simulink model "pointing_group24"  (R2023b)
settings: Solver=FixedStepAuto  StartTime=0.0  StopTime=T  RelTol=1e-3
values from neighbouring files (symbols this model uses):
  a = 6939    [Air_Drag_script.m]    (also in main.m = 6939.063; main_group24.m = 6978)
  AccMagn = 0.5    [main_group24.m]
  AccSunSens = 0.125    [main_group24.m]
  ARW = deg2rad(0.10)    [main_group24.m]
  by = 0.1    [main_group24.m]
  bz = 0.1    [main_group24.m]
  c = 2.99792*10^8    (= 299792000)    [main.m]    (also in main_group24.m = 299792458)
  Cd = 2.2    [main_group24.m]
  e = 0    [Air_Drag_script.m]    (also in main.m = 0.001304; main_group24.m)
  G = [gn, gm, gvali, gsvi]    [main.m]    (also in main_group24.m)
  GyroSampleRate = 10    [main_group24.m]
  H = [hn, hm, hvali, hsvi]    [main.m]    (also in main_group24.m)
  H_0 = ((g1_0^2)+(g1_1^2)+(h1_1^2))^0.5    (= 2.98059244128e-05)    [main_group24.m]
  i = deg2rad(97.5307)    [Air_Drag_script.m]    (also in main.m; main_group24.m = deg2rad(98))
  I_tot = [Ix 0 0; 0 Iy 0; 0 0 Iz]    [data_mass.m]    (also in main_group24.m)
  invI_tot = inv(I_tot)    [data_mass.m]    (also in main_group24.m)
  Ix = J(1,1)    [Air_Drag_script.m]    (also in data_mass.m = 0.0755003333333; main.m = 0.057749855; main_group24.m = 0.0755003333333)
  Iy = J(2,2)    [Air_Drag_script.m]    (also in data_mass.m = 0.0755003333333; main.m = 0.04143542; main_group24.m = 0.0755003333333)
  Iz = J(3,3)    [Air_Drag_script.m]    (also in data_mass.m = 0.055; main.m = 0.024624309; main_group24.m = 0.055)
  k1 = 5e-2    (= 0.05)    [main_group24.m]
  k2 = 2.5e-2    (= 0.025)    [main_group24.m]
  m = [0.1; 0.1; 0.1]    [main.m]    (also in main_group24.m)
  MB = [4; 0.1; 0.1; 0.3]    [main.m]    (also in main_group24.m)
  MMnoise = 15e-9*[1; 1; 1]    [main_group24.m]
  MMSampleRate = 1    [main_group24.m]
  mu = 3.98600433e+5    (= 398600.433)    [main.m]    (also in main_group24.m)
  n = 0.0011    [Air_Drag_script.m]    (also in main.m = sqrt(mu/a^3); main_group24.m = sqrt(mu/a^3))
  n_E = 729.2e-07    (= 7.292e-05)    [main_group24.m]
  om_E = 0.000072921    (= 7.2921e-05)    [main_group24.m]
  P = Fe/c    (= 4.52980041279e-06)    [main_group24.m]
  q0 = [ 1 1 1 1 ]'    [Air_Drag_script.m]    (also in main_group24.m = [0 0 0 1]')
  R_e = 6378    [main.m]    (also in main_group24.m)
  rho_air = 1.65e-13    [Air_Drag_script.m]    (also in main_group24.m = 6.967e-13)
  rho_d_body = 0.1*2/3    (= 0.0666666666667)    [main_group24.m]
  rho_d_sp = 0.1*2/3    (= 0.0666666666667)    [main_group24.m]
  rho_s_body = 0.5    [main_group24.m]
  rho_s_sp = 0.1    [main_group24.m]
  RRW = deg2rad(0.3)    [main_group24.m]
  SP = [1; 0.3; 0.1; 0.01]    [main.m]    (also in main_group24.m = [0.25; 0.1; 0.3; 0.01])
undefined symbols (not defined in the file or in its folder): pan, s1, s2, s3, s4, s5, s6, thrust
libraries: vrlib x25, matrix_library x17, simulink_extras x8, sharedutil x3, simulink x1
(part 1 of 5)
settings Model: Creator=hp  LastModifiedBy=adity

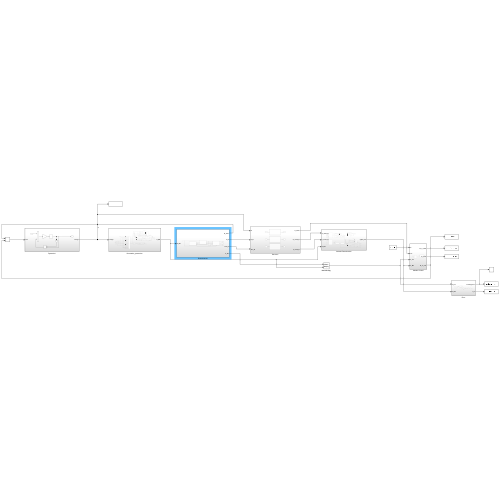
[thumbnail: Simulink's stored preview of the top-level diagram]
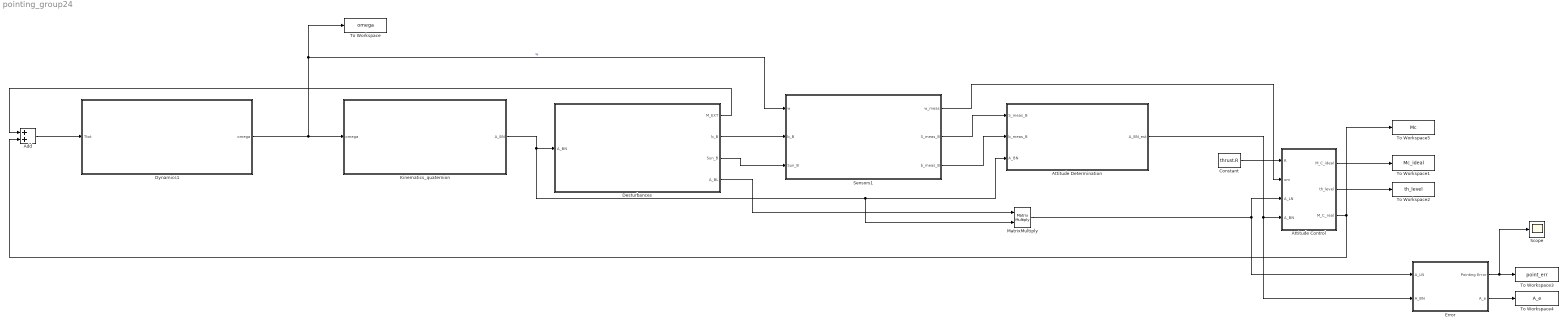
== system pointing_group24 ==
  Add : Sum
  Attitude Control : Subsystem
  Attitude Determination : Subsystem
  Constant : Constant  Value=thrust.R
  Desturbances : Subsystem
  Dynamics1 : Subsystem
  Error : Subsystem
  Kinematics_quaternion : Subsystem
  MatrixMultiply : Product  Multiplication=Matrix(*)
  Scope : Scope
  Sensors1 : Subsystem
  To Workspace : ToWorkspace  VariableName=omega  SaveFormat=Timeseries  SampleTime=-1
  To Workspace1 : ToWorkspace  VariableName=Mc_ideal  SaveFormat=Timeseries  SampleTime=-1
  To Workspace2 : ToWorkspace  VariableName=th_level  SaveFormat=Timeseries  SampleTime=-1
  To Workspace3 : ToWorkspace  VariableName=point_err  SaveFormat=Timeseries  SampleTime=-1
  To Workspace4 : ToWorkspace  VariableName=A_e  SaveFormat=Timeseries  SampleTime=-1
  To Workspace5 : ToWorkspace  VariableName=Mc  SaveFormat=Timeseries  SampleTime=-1
  wires:
  Add/1 -> Dynamics1/1(Ttot)
  Attitude Control/1(M_C_ideal) -> To Workspace1/1
  Attitude Control/2(th_level) -> To Workspace2/1
  Attitude Control/3(M_C_real) -> To Workspace5/1, Add/2
  Desturbances/2(b_B) -> Sensors1/2(b_B)
  Sensors1/2(S_meas_B) -> Attitude Determination/1(S_meas_B)
  Sensors1/1(w_meas) -> Attitude Control/2(om)
  Dynamics1/1(omega) -> Kinematics_quaternion/1(omega), To Workspace/1, Sensors1/1(w)  "w"
  Desturbances/1(M_EXT) -> Add/1
  Sensors1/3(b_meas_B) -> Attitude Determination/2(b_meas_B)
  Desturbances/3(Sun_B) -> Sensors1/3(Sun_B)
  Attitude Determination/1(A_BN_est) -> Error/2(A_BN), Attitude Control/4(A_BN)
  MatrixMultiply/1 -> Attitude Control/3(A_LN), Error/1(A_LN)
  Error/1(Pointing Error) -> Scope/1, To Workspace3/1
  Error/2(A_e) -> To Workspace4/1
  Constant/1 -> Attitude Control/1(R)
  Kinematics_quaternion/1(A_BN) -> MatrixMultiply/2, Attitude Determination/3(A_BN), Desturbances/1(A_BN)
  Desturbances/4(A_BL) -> MatrixMultiply/1

== system pointing_group24/Attitude Control ==
  R : Inport
  om : Inport  Port=2
  A_LN : Inport  Port=3
  A_BN : Inport  Port=4
  Constant : Constant  Value=[0;0;n]
  Ideal controller : Subsystem
  Reshape : Reshape  OutputDimensionality=Column vector (2-D)
  Thrusters : Subsystem
  M_C_ideal : Outport
  th_level : Outport  Port=2
  M_C_real : Outport  Port=3
  wires:
  Constant/1 -> Reshape/1
  Thrusters/3(th_level) -> th_level/1
  om/1 -> Ideal controller/1(om)
  Thrusters/1(M_C_real) -> M_C_real/1
  R/1 -> Thrusters/1(R)
  A_BN/1 -> Ideal controller/3(A_BN)
  Thrusters/2(M_C_ideal) -> M_C_ideal/1
  Ideal controller/1(S) -> Thrusters/2(S)
  Reshape/1 -> Ideal controller/4(om_des)
  A_LN/1 -> Ideal controller/2(A_des)

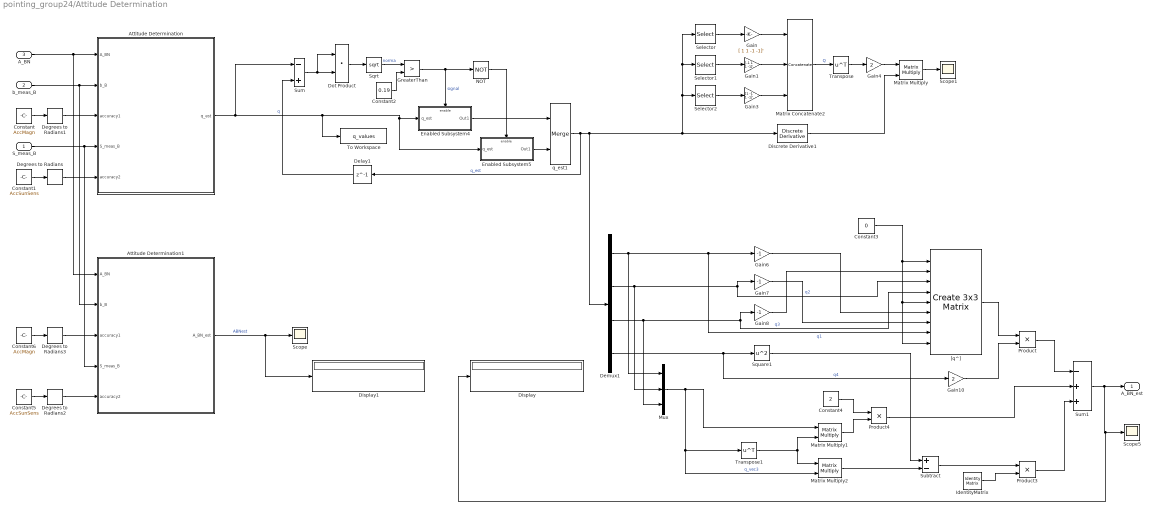
== system pointing_group24/Attitude Determination ==
  S_meas_B : Inport
  b_meas_B : Inport  Port=2
  A_BN : Inport  Port=3
  Attitude Determination : MATLAB Function  TreatAsAtomicUnit=on
  Attitude Determination1 : MATLAB Function  TreatAsAtomicUnit=on
  Constant : Constant  Value=AccMagn
  Constant1 : Constant  Value=AccSunSens
  Constant2 : Constant  Value=0.19
  Constant3 : Constant  Value=0
  Constant4 : Constant  Value=2
  Constant5 : Constant  Value=AccSunSens
  Constant6 : Constant  Value=AccMagn
  Degrees to Radians{,1..3} (4 alike) : simulink_extras/Transformations/Degrees to Radians
  Delay1 : Delay  DelayLength=1  InitialCondition=q0
  Demux1 : Demux
  Discrete Derivative1 : simulink/Discrete/Discrete Derivative  gainval=1.0  ICPrevScaledInput=0  OutMin=[]  OutMax=[]  OutDataType=fixdt(1, 16)  OutScaling=2^-10  DoSatur=off
  Display : Display
  Display1 : Display
  Dot Product : DotProduct  OutDataTypeStr=Inherit: Inherit via internal rule
  Enabled Subsystem4 : Subsystem  TreatAsAtomicUnit=on
  Enabled Subsystem5 : Subsystem  TreatAsAtomicUnit=on
  Gain : Gain  Gain=[ 1 1 -1 -1]'
  Gain1 : Gain  Gain=[-1 1 1 -1]'
  Gain10 : Gain  Gain=2
  Gain3 : Gain  Gain=[1 -1 1 -1]'
  Gain4 : Gain  Gain=2
  Gain6 : Gain  Gain=-1
  Gain7 : Gain  Gain=-1
  Gain8 : Gain  Gain=-1
  GreaterThan : RelationalOperator  Operator=>  OutDataTypeStr=boolean  RndMeth=Simplest  InputSameDT=off
  IdentityMatrix : IdentityMatrix  OutputDimensions=3
  Matrix Concatenate2 : Concatenate  NumInputs=3  Mode=Multidimensional array  ConcatenateDimension=2
  Matrix Multiply : Product  Multiplication=Matrix(*)
  Matrix Multiply1 : Product  Multiplication=Matrix(*)
  Matrix Multiply2 : Product  Multiplication=Matrix(*)
  Mux : Mux  Inputs=3
  NOT : Logic  Operator=NOT  IconShape=distinctive  AllPortsSameDT=off  OutDataTypeStr=boolean
  Product : Product
  Product3 : Product
  Product4 : Product
  Scope : Scope
  Scope1 : Scope
  Scope5 : Scope
  Selector : Selector  InputPortWidth=4  IndexOptions=Index vector (dialog)  Indices=[4 3 2 1]  OutputSizes=1
  Selector1 : Selector  InputPortWidth=4  IndexOptions=Index vector (dialog)  Indices=[3 4 1 2]  OutputSizes=1
  Selector2 : Selector  InputPortWidth=4  IndexOptions=Index vector (dialog)  Indices=[2 1 4 3]  OutputSizes=1
  Sqrt : Sqrt
  Square1 : Math  Operator=square
  Subtract : Sum  Inputs=+-
  Sum : Sum  Inputs=-+
  Sum1 : Sum  Inputs=-++
  To Workspace : ToWorkspace  VariableName=q_values  SaveFormat=Timeseries  SampleTime=-1
  Transpose : Math  Operator=transpose
  Transpose1 : Math  Operator=transpose
  "[q^]" : sharedutil/Create 3x3 Matrix  aMode=aMode
      settings: LibrarySourceBlock=aerolibutil/Create 3x3 Matrix
  q_est1 : Merge
  A_BN_est : Outport
  wires:
  b_meas_B/1 -> Attitude Determination1/2(b_B), Attitude Determination/2(b_B)
  S_meas_B/1 -> Attitude Determination1/4(S_meas_B), Attitude Determination/4(S_meas_B)
  Constant1/1 -> Degrees to Radians/1
  Constant/1 -> Degrees to Radians1/1
  A_BN/1 -> Attitude Determination1/1(A_BN), Attitude Determination/1(A_BN)
  Gain1/1 -> Matrix Concatenate2/2
  Matrix Multiply/1 -> Scope1/1
  Gain4/1 -> Matrix Multiply/1
  Gain/1 -> Matrix Concatenate2/1
  Selector/1 -> Gain/1
  Selector2/1 -> Gain3/1
  Transpose/1 -> Gain4/1
  Discrete Derivative1/1 -> Matrix Multiply/2
  Matrix Concatenate2/1 -> Transpose/1  "Q"
  Selector1/1 -> Gain1/1
  Gain3/1 -> Matrix Concatenate2/3
  Degrees to Radians1/1 -> Attitude Determination/3(accuracy1)
  Degrees to Radians/1 -> Attitude Determination/5(accuracy2)
  q_est1/1 -> Demux1/1, Selector1/1, Selector/1, Selector2/1, Discrete Derivative1/1, Delay1/1  "q_est"
  GreaterThan/1 -> NOT/1, Enabled Subsystem4/Enable  "signal"
  Enabled Subsystem5/1(Out1) -> q_est1/2
  Sum/1 -> Dot Product/1, Dot Product/2
  Delay1/1 -> Sum/2
  NOT/1 -> Enabled Subsystem5/Enable
  Enabled Subsystem4/1(Out1) -> q_est1/1
  Constant2/1 -> GreaterThan/2
  Sqrt/1 -> GreaterThan/1  "norma"
  Dot Product/1 -> Sqrt/1
  Attitude Determination/1(q_est) -> To Workspace/1, Enabled Subsystem4/1(q_est), Enabled Subsystem5/1(q_est), Sum/1  "q"
  "[q^]"/1 -> Product/1
  Square1/1 -> Subtract/1
  Matrix Multiply1/1 -> Product4/2
  Gain10/1 -> Product/2
  Sum1/1 -> Display/1, Scope5/1, A_BN_est/1
  Product/1 -> Sum1/1
  Gain8/1 -> "[q^]"/2
  Constant4/1 -> Product4/1
  Mux/1 -> Matrix Multiply1/1, Transpose1/1, Matrix Multiply2/2  "q_vec3"
  IdentityMatrix/1 -> Product3/2
  Transpose1/1 -> Matrix Multiply1/2, Matrix Multiply2/1
  Matrix Multiply2/1 -> Subtract/2
  Demux1/4 -> Gain10/1, Square1/1  "q4"
  Gain6/1 -> "[q^]"/6
  Demux1/2 -> Mux/2, Gain7/1, "[q^]"/3  "q2"
  Constant3/1 -> "[q^]"/5, "[q^]"/9, "[q^]"/1
  Gain7/1 -> "[q^]"/7
  Demux1/3 -> Mux/3, Gain8/1, "[q^]"/4  "q3"
  Product3/1 -> Sum1/3
  Product4/1 -> Sum1/2
  Demux1/1 -> Mux/1, Gain6/1, "[q^]"/8  "q1"
  Subtract/1 -> Product3/1
  Attitude Determination1/1(A_BN_est) -> Display1/1, Scope/1  "ABNest"
  Degrees to Radians2/1 -> Attitude Determination1/5(accuracy2)
  Constant5/1 -> Degrees to Radians2/1
  Degrees to Radians3/1 -> Attitude Determination1/3(accuracy1)
  Constant6/1 -> Degrees to Radians3/1

== system pointing_group24/Desturbances ==
  A_BN : Inport
  External Torques : Subsystem
      settings: PortSchema="{\"entries\":[{\"content\":{\"sides\":[{\"content\":{\"connectorIds\":[\"In1\",\"In2\",\"In3\",\"In4\",\"In5\"]},\"type\":\"ConnectorPlacement.EquallySpacedRectSide\",\"uuid\":\"8bd06876-b53a-4e9a-80a1-6b2ad32b6751\"},{\"content\":{\"connectorIds\":[\"Out1\",\"Out2\",\"Out3\"],\"side\":\"RIGHT\"},\"type\":\"ConnectorPlacement.EquallySpacedRectSide\",\"uuid\":\"d3d885b4-6948-49f2-a55d-d08402d43087\"},{\"content\":{\"side\":\"TOP\"},\"type\":\"ConnectorPlacement.EquallySpacedRectSide\",\"uuid\":\"3ccb2d92-0b83-4d3b-9d3e-c105f836e6c1\"},{\"content\":{\"connectorIds\":[\"In6\"],\"side\":\"BOTTOM\"},\"type\":\"ConnectorPlacement.EquallySpacedRectSide\",\"uuid\":\"856107a3-6a69-4cc1-b4e3-b2ecd550063c\"}]},\"type\":\"ConnectorPlacement.EquallySpacedConnector\",\"uuid\":\"94a3bf69-72fe-47a3-a305-62b7e77dc891\"}],\"packageUris\":[\"http://schema.mathworks.com/mf0/Connector/R2020b\"],\"version\":\"1.0\"}"
  Orbital Mechanics : Subsystem
  Relative Attitude : Subsystem
  M_EXT : Outport
  b_B : Outport  Port=2
  Sun_B : Outport  Port=3
  A_BL : Outport  Port=4
  wires:
  Relative Attitude/2(r_L) -> External Torques/2(r_L)
  A_BN/1 -> External Torques/5(A_BN), Relative Attitude/1(A_BN_ideal)
  Orbital Mechanics/1(theta) -> Relative Attitude/2(theta)
  Orbital Mechanics/2(r_N) -> Relative Attitude/3(r_N), External Torques/6(r_N)
  Orbital Mechanics/3(r) -> External Torques/3(r)
  External Torques/1(M_EXT) -> M_EXT/1
  External Torques/2(b_B) -> b_B/1
  External Torques/3(Sun_B) -> Sun_B/1
  Orbital Mechanics/4(v_rel_N) -> External Torques/4(v_rel_N)
  Relative Attitude/1(A_BL.) -> A_BL/1, External Torques/1(A_BL)

== system pointing_group24/Dynamics1 ==
  note: omega
  Ttot : Inport
  Add : Sum
  Cross Product : vrlib/Utilities/Cross Product
  Gain : Gain  Gain=invI_tot  Multiplication=Matrix(K*u)
  Gain1 : Gain  Gain=I_tot  Multiplication=Matrix(K*u)
  Integrator3 : Integrator  InitialCondition=[1e-3; 1e-3; 1e-3]  AbsoluteTolerance=10^-7
  omega : Outport
  wires:
  Gain1/1 -> Cross Product/1
  Ttot/1 -> Add/1
  Cross Product/1 -> Add/2
  Integrator3/1 -> omega/1, Cross Product/2, Gain1/1
  Gain/1 -> Integrator3/1
  Add/1 -> Gain/1

== system pointing_group24/Error ==
  A_LN : Inport
  A_BN : Inport  Port=2
  Acos1 : Trigonometry  Operator=acos
  Dot Product : DotProduct  OutDataTypeStr=Inherit: Inherit via internal rule
  Product : Product  Multiplication=Matrix(*)
  Product1 : Product  Multiplication=Matrix(*)
  Radians to Degrees1 : simulink_extras/Transformations/Radians to Degrees
  Transpose : Math  Operator=transpose
  z_B : Constant  Value=[0;0;1]
  z_L : Constant  Value=[0;0;1]
  Pointing Error : Outport
  A_e : Outport  Port=2
  wires:
  A_LN/1 -> Transpose/1
  A_BN/1 -> Product/1
  Transpose/1 -> Product/2
  Product/1 -> Product1/1, A_e/1  "A_BL"
  Radians to Degrees1/1 -> Pointing Error/1
  z_L/1 -> Product1/2
  Dot Product/1 -> Acos1/1
  Acos1/1 -> Radians to Degrees1/1
  Product1/1 -> Dot Product/1  "x_L_B"
  z_B/1 -> Dot Product/2

== system pointing_group24/Kinematics_quaternion ==
  omega : Inport
  Constant : Constant  Value=0
  Constant1 : Constant  Value=0
  Constant2 : Constant  Value=2
  Demux : Demux  Outputs=3
  Demux1 : Demux
  Divide : Product  Inputs=/*
  Dot Product : DotProduct  OutDataTypeStr=Inherit: Inherit via internal rule
  Gain{1..3,6..8} (6 alike) : Gain  Gain=-1
  Gain10 : Gain  Gain=2
  Gain9 : Gain  Gain=1/2
  IdentityMatrix : IdentityMatrix  OutputDimensions=3
  Integrator : Integrator  InitialCondition=q0
  Matrix Multiply : Product  Multiplication=Matrix(*)
  Matrix Multiply1 : Product  Multiplication=Matrix(*)
  Matrix Multiply2 : Product  Multiplication=Matrix(*)
  Mux : Mux  Inputs=3
  OMEGA : Concatenate  NumInputs=16  Mode=Multidimensional array  ConcatenateDimension=2
  Product : Product
  Product3 : Product
  Product4 : Product
  Reshape : Reshape  OutputDimensionality=Customize  OutputDimensions=[4,4]
  Scope : Scope
  Scope5 : Scope
  Square Root2 : Sqrt
  Square1 : Math  Operator=square
  Subtract : Sum  Inputs=+-
  Sum : Sum  Inputs=-++
  Transpose : Math  Operator=transpose
  "[q^]" : sharedutil/Create 3x3 Matrix  aMode=aMode
      settings: LibrarySourceBlock=aerolibutil/Create 3x3 Matrix
  A_BN : Outport
  wires:
  Matrix Multiply/1 -> Gain9/1
  Square Root2/1 -> Divide/1
  Constant/1 -> OMEGA/16, OMEGA/11, OMEGA/6, OMEGA/1
  Integrator/1 -> Dot Product/1, Dot Product/2, Divide/2  "q"
  OMEGA/1 -> Reshape/1
  Constant1/1 -> "[q^]"/5, "[q^]"/9, "[q^]"/1
  Demux1/1 -> Mux/1, Gain6/1, "[q^]"/8  "q1"
  Demux1/2 -> Mux/2, Gain7/1, "[q^]"/3  "q2"
  Demux1/4 -> Gain10/1, Square1/1  "q4"
  Gain8/1 -> "[q^]"/2
  Gain6/1 -> "[q^]"/6
  Gain7/1 -> "[q^]"/7
  Transpose/1 -> Matrix Multiply1/2, Matrix Multiply2/1
  Gain10/1 -> Product/2
  "[q^]"/1 -> Product/1
  Square1/1 -> Subtract/1
  Matrix Multiply2/1 -> Subtract/2
  Divide/1 -> Scope/1, Demux1/1, Matrix Multiply/2  "q"
  Subtract/1 -> Product3/1
  IdentityMatrix/1 -> Product3/2
  Product/1 -> Sum/1
  Product3/1 -> Sum/3
  Constant2/1 -> Product4/1
  Matrix Multiply1/1 -> Product4/2
  Product4/1 -> Sum/2
  Demux1/3 -> Mux/3, Gain8/1, "[q^]"/4  "q3"
  Mux/1 -> Matrix Multiply1/1, Transpose/1, Matrix Multiply2/2  "q_vec3"
  Sum/1 -> Scope5/1, A_BN/1
  Dot Product/1 -> Square Root2/1
  Reshape/1 -> Matrix Multiply/1
  Gain9/1 -> Integrator/1  "q_dot"
  omega/1 -> Demux/1
  Demux/1 -> OMEGA/7, OMEGA/4, Gain2/1  "wx"
  Demux/2 -> OMEGA/8, OMEGA/9, Gain3/1  "wy"
  Demux/3 -> OMEGA/2, OMEGA/12, Gain1/1  "wz"
  Gain3/1 -> OMEGA/3, OMEGA/14
  Gain1/1 -> OMEGA/5, OMEGA/15
  Gain2/1 -> OMEGA/13, OMEGA/10

== system pointing_group24/Sensors1 ==
  w : Inport
  b_B : Inport  Port=2
  Sun_B : Inport  Port=3
  Gyroscope : Subsystem
  Magnetometer : Subsystem
  Sun Sensor : Subsystem
  w_meas : Outport
  S_meas_B : Outport  Port=2
  b_meas_B : Outport  Port=3
  wires:
  w/1 -> Gyroscope/1(w)
  Gyroscope/1(w_meas) -> w_meas/1
  Sun Sensor/1(S_meas_B) -> S_meas_B/1
  Sun_B/1 -> Sun Sensor/1(Sun_B)
  b_B/1 -> Magnetometer/1(b_B)
  Magnetometer/1(b_meas_B) -> b_meas_B/1

== system pointing_group24/Attitude Control/Ideal controller ==
  om : Inport
  A_des : Inport  Port=2
  A_BN : Inport  Port=3
  om_des : Inport  Port=4
  Constant : Constant  Value=[0 0 0]'
  Cross Product : vrlib/Utilities/Cross Product
  Gain : Gain  Gain=I_tot  Multiplication=Matrix(K*u) (u vector)
  Gain1 : Gain  Gain=k1
  Gain2 : Gain  Gain=k2
  Gain4 : Gain  Gain=I_tot  Multiplication=Matrix(K*u) (u vector)
  Gain5 : Gain  Gain=I_tot  Multiplication=Matrix(K*u) (u vector)
  MATLAB Function : MATLAB Function  TreatAsAtomicUnit=on
  Matrix Multiply{1..5} (5 alike) : Product  Multiplication=Matrix(*)
  Subsystem2 : Subsystem
  Sum : Sum
  Sum1 : Sum  Inputs=+-
  Sum2 : Sum  Inputs=-+-
  Sum3 : Sum
  Transpose : Math  Operator=transpose
  S : Outport
  wires:
  Gain1/1 -> Sum/1
  om/1 -> Cross Product/1, Gain/1, Sum1/1
  Matrix Multiply1/1 -> Matrix Multiply2/1, Matrix Multiply5/1, Matrix Multiply3/1, MATLAB Function/1(A)  "A_e"
  Sum1/1 -> Subsystem2/1(om), Gain1/1  "om_e"
  Cross Product/1 -> Sum2/1
  Subsystem2/1(om^) -> Matrix Multiply4/1
  Matrix Multiply2/1 -> Sum1/2
  Matrix Multiply3/1 -> Matrix Multiply4/2
  Gain/1 -> Cross Product/2
  MATLAB Function/1(Av) -> Gain2/1
  Transpose/1 -> Matrix Multiply1/2
  A_BN/1 -> Matrix Multiply1/1
  Sum2/1 -> Sum3/2
  Matrix Multiply4/1 -> Gain4/1
  Matrix Multiply5/1 -> Gain5/1
  A_des/1 -> Transpose/1
  om_des/1 -> Matrix Multiply2/2, Matrix Multiply3/2
  Gain2/1 -> Sum/2
  Sum/1 -> Sum3/1
  Gain4/1 -> Sum2/2
  Gain5/1 -> Sum2/3
  Sum3/1 -> S/1
  Constant/1 -> Matrix Multiply5/2

== system pointing_group24/Attitude Control/Thrusters ==
  R : Inport
  S : Inport  Port=2
  Constant : Constant  Value=thrust.w
  Constant1 : Constant  Value=thrust.T_min
  Constant2 : Constant  Value=thrust.T_max
  Divide : Product  Inputs=*/
  Ideal Control Torque : Subsystem
  MATLAB Function1 : MATLAB Function  TreatAsAtomicUnit=on
  MATLAB Function2 : MATLAB Function  TreatAsAtomicUnit=on
  Matrix Multiply : Product  Multiplication=Matrix(*)
  Matrix Multiply1 : Product  Multiplication=Matrix(*)
  Max of Elements : MinMax  Function=max  ZeroCross=off
  Product : Product
  R1 : InportShadow
  Sum : Sum
  M_C_real : Outport
  M_C_ideal : Outport  Port=2
  th_level : Outport  Port=3
  wires:
  MATLAB Function2/2(th_level) -> th_level/1
  Sum/1 -> MATLAB Function2/1(u_c)  "real"
  Matrix Multiply/1 -> Sum/1, Divide/1
  R1/1 -> Matrix Multiply1/1
  Matrix Multiply1/1 -> M_C_real/1
  MATLAB Function1/1(y) -> Matrix Multiply/1
  R/1 -> MATLAB Function1/1(u)
  Ideal Control Torque/1(M_C_ideal) -> M_C_ideal/1, Matrix Multiply/2
  Max of Elements/1 -> Product/1  "gamma"
  Divide/1 -> Max of Elements/1
  Product/1 -> Sum/2
  Constant/1 -> Product/2, Divide/2  "w"
  MATLAB Function2/1(u_c_real) -> Matrix Multiply1/2  "real"
  S/1 -> Ideal Control Torque/1(S)
  Constant1/1 -> MATLAB Function2/2(T_min)
  Constant2/1 -> MATLAB Function2/3(T_max)

== system pointing_group24/Attitude Determination/Enabled Subsystem4 ==
  q_est : Inport
  Enable : EnablePort
  Gain : Gain  Gain=-1
  Out1 : Outport
  wires:
  q_est/1 -> Gain/1
  Gain/1 -> Out1/1

== system pointing_group24/Attitude Determination/Enabled Subsystem5 ==
  q_est : Inport
  Enable : EnablePort
  Out1 : Outport
  wires:
  q_est/1 -> Out1/1

== system pointing_group24/Desturbances/External Torques ==
  A_BL : Inport
  r_L : Inport  Port=2
  r : Inport  Port=3
  v_rel_N : Inport  Port=4
  A_BN : Inport  Port=5
  r_N : Inport  Port=6
  Air Drag : Subsystem
  Constant : Constant  Value=MB
  Constant1 : Constant  Value=SP
  Constant2 : Constant  Value=MB
  Constant3 : Constant  Value=SP
  M_GG : Subsystem
  Mag field senza fcn : Subsystem
  Magnetic field : Subsystem
  MatrixMultiply : Product  Multiplication=Matrix(*)
  Reflected radiation : Subsystem
  SRP con frecce : Subsystem
  Scope{,1..6} (7 alike) : Scope
  Solar radiation : Subsystem
  Sum of Elements : Sum  Inputs=++++
  Sun position : Subsystem
  To Workspace : ToWorkspace  VariableName=M_GG  SaveFormat=Timeseries  SampleTime=-1
  To Workspace1 : ToWorkspace  VariableName=M_SRP  SaveFormat=Timeseries  SampleTime=-1
  To Workspace2 : ToWorkspace  VariableName=M_MAG  SaveFormat=Timeseries  SampleTime=-1
  M_EXT : Outport
  b_B : Outport  Port=2
  Sun_B : Outport  Port=3
  wires:
  r/1 -> M_GG/2(r)
  Constant/1 -> Solar radiation/2(MB)
  Constant1/1 -> Solar radiation/3(SP)
  A_BN/1 -> Reflected radiation/1(A_BN), Solar radiation/1(A_BN), Magnetic field/2(A_BN), MatrixMultiply/1, Mag field senza fcn/2(A_BN), Sun position/1(A_BN)
  Magnetic field/1(M_MAG) -> Scope2/1, Sum of Elements/3, To Workspace2/1
  Sum of Elements/1 -> M_EXT/1
  A_BL/1 -> M_GG/1(A_BL)
  r_L/1 -> Magnetic field/1(r_L)
  M_GG/1(M_GG1) -> Scope/1, Sum of Elements/1, To Workspace/1
  Solar radiation/1(T_SRP) -> Scope1/1, To Workspace1/1, Sum of Elements/2
  Magnetic field/2(b_B) -> b_B/1
  Solar radiation/2(Sun_B) -> Sun_B/1
  Sun position/1(S_B) -> SRP con frecce/1(S_B)
  Mag field senza fcn/1(T_mag) -> Scope3/1
  MatrixMultiply/1 -> Air Drag/1(v_rel_B)
  Air Drag/1(Tair) -> Scope4/1, Sum of Elements/4
  SRP con frecce/1(Tsrp) -> Scope5/1
  r_N/1 -> Reflected radiation/4(r_N), Mag field senza fcn/1(r_N)
  v_rel_N/1 -> MatrixMultiply/2, Air Drag/2(v_rel_N^2)
  Constant3/1 -> Reflected radiation/3(SP)
  Constant2/1 -> Reflected radiation/2(MB)
  Reflected radiation/1(T_reflect) -> Scope6/1

== system pointing_group24/Desturbances/Orbital Mechanics ==
  Sat Position magnitude : Subsystem
  Sat True Anomaly : Subsystem
  Sat pos & rel vel vectors in inertial frame : Subsystem
  Scope : Scope
  theta : Outport
  r_N : Outport  Port=2
  r : Outport  Port=3
  v_rel_N : Outport  Port=4
  wires:
  Sat True Anomaly/1(theta) -> Sat pos & rel vel vectors in inertial frame/2(theta), theta/1, Sat Position magnitude/1(theta)  "theta"
  Sat Position magnitude/1(r) -> Scope/1, r/1, Sat pos & rel vel vectors in inertial frame/1(r)
  Sat pos & rel vel vectors in inertial frame/1(r_N) -> r_N/1  "r_N"
  Sat pos & rel vel vectors in inertial frame/2(v_rel_N) -> v_rel_N/1

== system pointing_group24/Desturbances/Relative Attitude ==
  A_BN_ideal : Inport
  theta : Inport  Port=2
  r_N : Inport  Port=3
  A_BL : Subsystem
  A_LN : Subsystem
  MatrixMultiply : Product  Multiplication=Matrix(*)
  A_BL. : Outport
  r_L : Outport  Port=2
  wires:
  A_LN/1(A_LN) -> MatrixMultiply/1, A_BL/2(A_LN)
  theta/1 -> A_LN/1(theta)
  A_BN_ideal/1 -> A_BL/1(A_BN)
  A_BL/1(A_BL) -> A_BL./1
  r_N/1 -> MatrixMultiply/2
  MatrixMultiply/1 -> r_L/1

== system pointing_group24/Sensors1/Gyroscope ==
  w : Inport
  ARW : RandomNumber  Variance=(deg2rad(ARW)/sqrt(3600)/sqrt(1/GyroSampleRate))^2*[1;1;1]  SampleTime=1/GyroSampleRate
  Integrator : Integrator
  RRW : RandomNumber  Variance=(deg2rad(RRW)/3600/sqrt(1/GyroSampleRate))^2* [1;1;1]  SampleTime=1/GyroSampleRate
  Sum : Sum  Inputs=+++
  w_meas : Outport
  wires:
  RRW/1 -> Integrator/1  "b_dot"
  ARW/1 -> Sum/2  "n"
  Integrator/1 -> Sum/3  "b"
  Sum/1 -> w_meas/1
  w/1 -> Sum/1

== system pointing_group24/Sensors1/Magnetometer ==
  b_B : Inport
  Constant : Constant  Value=MMnoise
  MatrixMultiply : Product  Multiplication=Matrix(*)
  Subsystem : Subsystem
  Sum : Sum
  b_meas_B : Outport
  wires:
  Constant/1 -> Sum/2
  b_B/1 -> Sum/1  "b_B"
  Subsystem/1(A_epsMM) -> MatrixMultiply/1
  Sum/1 -> MatrixMultiply/2
  MatrixMultiply/1 -> b_meas_B/1

== system pointing_group24/Sensors1/Sun Sensor ==
  Sun_B : Inport
  Matrix Multiply1 : Product  Multiplication=Matrix(*)
  Subsystem : Subsystem
  S_meas_B : Outport
  wires:
  Sun_B/1 -> Matrix Multiply1/2
  Subsystem/1(A_eps) -> Matrix Multiply1/1  "A_eps"
  Matrix Multiply1/1 -> S_meas_B/1

== system pointing_group24/Attitude Control/Ideal controller/Subsystem2 ==
  om : Inport
  Constant : Constant  Value=0
  Demux : Demux  Outputs=3
  Gain : Gain  Gain=-1
  Gain1 : Gain  Gain=-1
  Gain2 : Gain  Gain=-1
  Subsystem : Subsystem
  om^ : Outport
  wires:
  Demux/2 -> Subsystem/3(A13), Gain2/1
  Demux/3 -> Subsystem/4(A21), Gain/1
  Gain2/1 -> Subsystem/7(A31)
  Gain/1 -> Subsystem/2(A12)
  Subsystem/1(A_BN_312) -> om^/1
  Constant/1 -> Subsystem/1(A11), Subsystem/5(A22), Subsystem/9(A33)
  Demux/1 -> Subsystem/8(A32), Gain1/1
  Gain1/1 -> Subsystem/6(A23)
  om/1 -> Demux/1

== system pointing_group24/Attitude Control/Thrusters/Ideal Control Torque ==
  S : Inport
  Constant : Constant  Value=thrust.T_min
  Constant1 : Constant  Value=thrust.T_max
  Constant4 : Constant  Value=[bz;bz;by]
  Gain3 : Gain  Gain=-1
  MATLAB Function2 : MATLAB Function  TreatAsAtomicUnit=on
  Matrix Multiply : Product
  Product2 : Product
  Sign : Signum
  M_C_ideal : Outport
  wires:
  S/1 -> Sign/1, MATLAB Function2/1(S)
  Product2/1 -> Gain3/1
  Gain3/1 -> M_C_ideal/1
  Matrix Multiply/1 -> Product2/1
  MATLAB Function2/1(T) -> Matrix Multiply/2
  Sign/1 -> Product2/2
  Constant4/1 -> Matrix Multiply/1
  Constant/1 -> MATLAB Function2/2(T_min)
  Constant1/1 -> MATLAB Function2/3(T_max)

== system pointing_group24/Desturbances/External Torques/Air Drag ==
  v_rel_B : Inport
  v_rel_N^2 : Inport  Port=2
  Dot Product : DotProduct  OutDataTypeStr=Inherit: Inherit via internal rule
  Gain : Gain  Gain=4
  Gain1 : Gain  Gain=4
  Normalize Vector1 : vrlib/Utilities/Normalize Vector  maxzero=0
  Subsystem : Subsystem
  Subsystem1 : Subsystem
  Subsystem2 : Subsystem
  Subsystem3 : Subsystem
  Subsystem4 : Subsystem
  Subsystem5 : Subsystem
  Subsystem6 : Subsystem
  Subsystem7 : Subsystem
  Sum : Sum  Inputs=++++++++
  Tair : Outport
  wires:
  v_rel_B/1 -> Normalize Vector1/1
  Sum/1 -> Tair/1
  Subsystem/1(Pan1) -> Sum/1
  Subsystem1/1(Pan2) -> Sum/2
  Subsystem2/1(Pan3) -> Sum/3
  Subsystem3/1(Pan4) -> Sum/4
  Subsystem4/1(Pan5) -> Sum/5
  Subsystem5/1(Pan6) -> Sum/6
  Subsystem6/1(Ps1) -> Gain1/1
  Subsystem7/1(Ps2) -> Gain/1
  Gain/1 -> Sum/8
  Gain1/1 -> Sum/7
  Normalize Vector1/1 -> Subsystem1/2(v_rel_B), Subsystem2/2(v_rel_B), Subsystem3/2(v_rel_B), Subsystem4/2(v_rel_B), Subsystem5/2(v_rel_B), Subsystem6/2(v_rel_B), Subsystem7/2(v_rel_B), Subsystem/2(v_rel_B)
  v_rel_N^2/1 -> Dot Product/2, Dot Product/1
  Dot Product/1 -> Subsystem/1(v_rel_N^2), Subsystem1/1(v_rel_N^2), Subsystem2/1(v_rel_N^2), Subsystem3/1(v_rel_N^2), Subsystem4/1(v_rel_N^2), Subsystem5/1(v_rel_N^2), Subsystem6/1(v_rel_N^2), Subsystem7/1(v_rel_N^2)

== system pointing_group24/Desturbances/External Torques/M_GG ==
  A_BL : Inport
  r : Inport  Port=2
  GG Torque1 : Subsystem
  "c1, c2, c3" : Subsystem
  M_GG1 : Outport
  wires:
  A_BL/1 -> "c1, c2, c3"/1(A_BL)
  "c1, c2, c3"/1(c1) -> GG Torque1/1(c1)
  "c1, c2, c3"/2(c2) -> GG Torque1/2(c2)
  "c1, c2, c3"/3(c3) -> GG Torque1/3(c3)
  r/1 -> GG Torque1/4(r)
  GG Torque1/1(M_GG) -> M_GG1/1

== system pointing_group24/Desturbances/External Torques/Mag field senza fcn ==
  r_N : Inport
  A_BN : Inport  Port=2
  Add : Sum  Inputs=-+
  Clock : Clock
  Constant : Constant  Value=11.5
  Constant1 : Constant  Value=n_E
  Constant2 : Constant  Value=H_0
  Constant3 : Constant  Value=R_e
  Constant4 : Constant  Value=3
  Constant5 : Constant  Value=3
  Constant6 : Constant  Value=3
  Constant7 : Constant  Value=m
  Cos : Trigonometry  Operator=cos
  Cos1 : Trigonometry  Operator=cos
  Cross Product : vrlib/Utilities/Cross Product
  Degrees to Radians : simulink_extras/Transformations/Degrees to Radians
  Divide : Product  Inputs=/*
  Dot Product : DotProduct  OutDataTypeStr=Inherit: Inherit via internal rule
  Dot Product1 : DotProduct  OutDataTypeStr=Inherit: Inherit via internal rule
  Gain : Gain  Gain=-1
  MatrixMultiply : Product  Multiplication=Matrix(*)
  Mux : Mux  Inputs=3
  Normalize Vector : vrlib/Utilities/Normalize Vector  maxzero=0
  Power : Math  Operator=pow
  Power1 : Math  Operator=pow
  Product{,1..6} (7 alike) : Product
  Scope : Scope
  Sin : Trigonometry
  Sin1 : Trigonometry
  Sqrt : Sqrt
  T_mag : Outport
  wires:
  Constant/1 -> Degrees to Radians/1
  Constant1/1 -> Product/1
  Clock/1 -> Product/2
  Product/1 -> Sin1/1, Cos/1
  Sin/1 -> Product2/1, Product1/1
  Cos/1 -> Product1/2
  Sin1/1 -> Product2/2
  Product1/1 -> Mux/1
  Cos1/1 -> Mux/3
  Product2/1 -> Mux/2
  Constant4/1 -> Power/2
  Constant3/1 -> Power/1
  Constant5/1 -> Power1/2
  Constant2/1 -> Product3/1
  Power/1 -> Product3/2
  r_N/1 -> Dot Product/2, Dot Product/1, Normalize Vector/1
  Dot Product/1 -> Sqrt/1
  Sqrt/1 -> Power1/1
  Mux/1 -> Gain/1
  Normalize Vector/1 -> Product4/2, Dot Product1/2
  Dot Product1/1 -> Product4/1
  Constant6/1 -> Product5/1
  Product4/1 -> Product5/2
  Product6/1 -> MatrixMultiply/2
  A_BN/1 -> MatrixMultiply/1
  MatrixMultiply/1 -> Cross Product/2
  Constant7/1 -> Cross Product/1
  Cross Product/1 -> Scope/1, T_mag/1
  Product5/1 -> Add/2
  Power1/1 -> Divide/1
  Product3/1 -> Divide/2
  Add/1 -> Product6/1
  Divide/1 -> Product6/2
  Degrees to Radians/1 -> Cos1/1, Sin/1
  Gain/1 -> Dot Product1/1, Add/1

== system pointing_group24/Desturbances/External Torques/Magnetic field ==
  r_L : Inport
  A_BN : Inport  Port=2
  Clock : Clock
  Constant : Constant  Value=m
  Constant1 : Constant  Value=R_e*1000
  Constant3 : Constant  Value=G
  Constant4 : Constant  Value=H
  Cross Product1 : matrix_library/Cross Product
  MATLAB Function : MATLAB Function  TreatAsAtomicUnit=on
  MatrixMultiply : Product  Multiplication=Matrix(*)
  Normalize Vector : vrlib/Utilities/Normalize Vector  maxzero=0
  Reshape1 : Reshape  OutputDimensionality=Column vector (2-D)
  M_MAG : Outport
  b_B : Outport  Port=2
  wires:
  Constant1/1 -> MATLAB Function/2(r)
  Clock/1 -> MATLAB Function/3(t)
  Constant3/1 -> MATLAB Function/4(G)
  MATLAB Function/1(b_N) -> Reshape1/1
  r_L/1 -> MATLAB Function/1(r_LVLH)
  Reshape1/1 -> MatrixMultiply/2
  Constant4/1 -> MATLAB Function/5(H)
  A_BN/1 -> MatrixMultiply/1
  Constant/1 -> Cross Product1/1
  MatrixMultiply/1 -> Normalize Vector/1, Cross Product1/2
  Cross Product1/1 -> M_MAG/1
  Normalize Vector/1 -> b_B/1

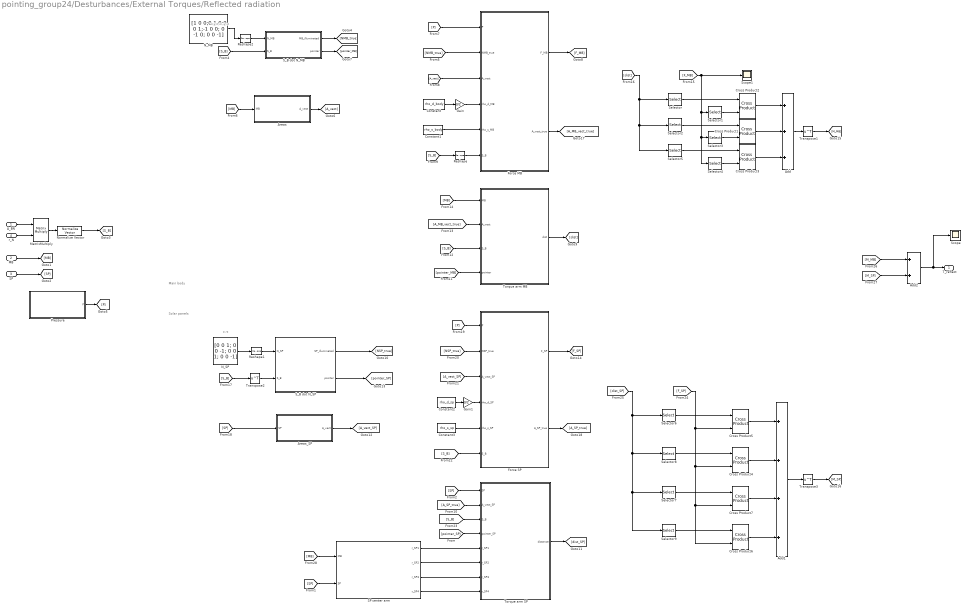
== system pointing_group24/Desturbances/External Torques/Reflected radiation ==
  note: Solar panels
  note: z,-z
  note: x,y,z,-x,-y,-z
  note: Main body
  A_BN : Inport
  MB : Inport  Port=2
  SP : Inport  Port=3
  r_N : Inport  Port=4
  Add : Sum  Inputs=3
  Add1 : Sum  Inputs=++++
  Add2 : Sum
  Areas : Subsystem
  Areas_SP : Subsystem
  Constant : Constant  Value=rho_d_body
  Constant1 : Constant  Value=rho_s_body
  Constant2 : Constant  Value=rho_d_sp
  Constant3 : Constant  Value=rho_s_sp
  Cross Product{1..7} (7 alike) : matrix_library/Cross Product
  Force MB : Subsystem
  Force SP : Subsystem
  Gain : Gain  Gain=3/2
  Gain1 : Gain  Gain=3/2
  MatrixMultiply : Product  Multiplication=Matrix(*)
  N_MB : Constant  Value=[1 0 0;0 1 0;0 0 1;-1 0 0; 0 -1 0; 0 0 -1]  VectorParams1D=off
  N_SP : Constant  Value=[0 0 1; 0 0 -1; 0 0 1; 0 0 -1]  VectorParams1D=off
  Normalize Vector : vrlib/Utilities/Normalize Vector  maxzero=0
  Pressure : Subsystem
  Reshape : Reshape  OutputDimensionality=Column vector (2-D)
  Reshape1 : Reshape  OutputDimensionality=Customize  OutputDimensions=[4,3]
  Reshape2 : Reshape  OutputDimensionality=Customize  OutputDimensions=[6,3]
  SP center arm : Subsystem
  S_B dot N_MB : Subsystem
  S_B dot N_SP : Subsystem
  Scope : Scope
  Scope1 : Scope
  Selector : Selector  NumberOfDimensions=2  InputPortWidth=3  IndexOptions=Index vector (dialog),Index vector (dialog)  Indices=1,[1 2 3]  OutputSizes=1,1
  Selector1 : Selector  NumberOfDimensions=2  InputPortWidth=3  IndexOptions=Index vector (dialog),Index vector (dialog)  Indices=1,[1 2 3]  OutputSizes=1,1
  Selector2 : Selector  NumberOfDimensions=2  InputPortWidth=3  IndexOptions=Index vector (dialog),Index vector (dialog)  Indices=2,[1 2 3]  OutputSizes=1,1
  Selector3 : Selector  NumberOfDimensions=2  InputPortWidth=3  IndexOptions=Index vector (dialog),Index vector (dialog)  Indices=2,[1 2 3]  OutputSizes=1,1
  Selector4 : Selector  NumberOfDimensions=2  InputPortWidth=3  IndexOptions=Index vector (dialog),Index vector (dialog)  Indices=3,[1 2 3]  OutputSizes=1,1
  Selector5 : Selector  NumberOfDimensions=2  InputPortWidth=3  IndexOptions=Index vector (dialog),Index vector (dialog)  Indices=3,[1 2 3]  OutputSizes=1,1
  Selector6 : Selector  NumberOfDimensions=2  InputPortWidth=3  IndexOptions=Index vector (dialog),Index vector (dialog)  Indices=1,[1 2 3]  OutputSizes=1,1
  Selector7 : Selector  NumberOfDimensions=2  InputPortWidth=3  IndexOptions=Index vector (dialog),Index vector (dialog)  Indices=3,[1 2 3]  OutputSizes=1,1
  Selector8 : Selector  NumberOfDimensions=2  InputPortWidth=3  IndexOptions=Index vector (dialog),Index vector (dialog)  Indices=2,[1 2 3]  OutputSizes=1,1
  Selector9 : Selector  NumberOfDimensions=2  InputPortWidth=3  IndexOptions=Index vector (dialog),Index vector (dialog)  Indices=4,[1 2 3]  OutputSizes=1,1
  Torque arm MB : Subsystem
  Torque arm SP : Subsystem
  Transpose1 : Math  Operator=transpose
  Transpose2 : Math  Operator=transpose
  Transpose3 : Math  Operator=transpose
  T_reflect : Outport
  wires:
  Cross Product7/1 -> Add1/3
  Cross Product6/1 -> Add1/4
  [F_SP] -> Cross Product4/2, Cross Product7/2, Cross Product6/2, Cross Product5/2
  [dist_SP] -> Selector8/1, Selector7/1, Selector9/1, Selector6/1
  Selector9/1 -> Cross Product6/1
  Selector7/1 -> Cross Product7/1
  SP center arm/4(r_SP4) -> Torque arm SP/8(r_SP4)
  SP center arm/3(r_SP3) -> Torque arm SP/7(r_SP3)
  Gain1/1 -> Force SP/4(rho_d_SP)
  Gain/1 -> Force MB/4(rho_d_MB)
  SP center arm/2(r_SP2) -> Torque arm SP/6(r_SP2)
  SP center arm/1(r_SP1) -> Torque arm SP/5(r_SP1)
  [MB] -> SP center arm/1(MB)
  [SP] -> SP center arm/2(SP)
  Cross Product3/1 -> Add/3
  [SP] -> Torque arm SP/1(SP)
  [M_SP] -> Add2/2
  Cross Product1/1 -> Add/2
  Selector5/1 -> Cross Product3/1
  Selector6/1 -> Cross Product5/1
  S_B dot N_SP/1(SP_illuminated) -> [NSP_true]
  Force SP/1(F_SP) -> [F_SP]
  Cross Product2/1 -> Add/1
  Reshape/1 -> Force MB/6(S_B)
  [A_vect_SP] -> Force SP/3(A_vect_SP)
  Cross Product5/1 -> Add1/1
  [S_B] -> Transpose2/1
  [S_B] -> Force SP/6(S_B)
  Selector3/1 -> Cross Product1/2
  Add2/1 -> T_reflect/1, Scope/1
  [pointer_MB] -> Torque arm MB/4(pointer)
  Force MB/2(A_vect_true) -> [A_MB_vect_true]
  S_B dot N_MB/2(pointer) -> [pointer_MB]
  Selector4/1 -> Cross Product3/2
  SP/1 -> [SP]
  [S_B] -> Torque arm SP/3(S_B)
  Force SP/2(A_SP_true) -> [A_SP_true]
  [S_B] -> Torque arm MB/3(S_B)
  N_SP/1 -> Reshape1/1
  [NSP_true] -> Force SP/2(NSP_true)
  [dist] -> Selector/1, Selector5/1, Selector2/1
  Selector8/1 -> Cross Product4/1
  Constant/1 -> Gain/1
  Constant2/1 -> Gain1/1
  Normalize Vector/1 -> [S_B]
  Pressure/1(P) -> [P]
  [A_MB_vect_true] -> Torque arm MB/2(A_vect)
  Constant1/1 -> Force MB/5(rho_s_MB)
  Selector1/1 -> Cross Product2/2
  [A_vect] -> Force MB/3(A_vect)
  [P] -> Force SP/1(P)
  [S_B] -> Reshape/1
  Selector/1 -> Cross Product2/1
  Force MB/1(F_MB) -> [F_MB]
  S_B dot N_SP/2(pointer) -> [pointer_SP]
  Torque arm MB/1(dist) -> [dist]
  Reshape2/1 -> S_B dot N_MB/1(N_MB)
  Torque arm SP/1(distance) -> [dist_SP]
  Add/1 -> Transpose1/1
  [A_SP_true] -> Torque arm SP/2(A_vect_SP)
  [SP] -> Areas_SP/1(SP)
  Transpose2/1 -> S_B dot N_SP/2(S_B)
  Add1/1 -> Transpose3/1
  A_BN/1 -> MatrixMultiply/1
  [F_MB] -> Selector1/1, Selector3/1, Selector4/1, Scope1/1
  Cross Product4/1 -> Add1/2
  [pointer_SP] -> Torque arm SP/4(pointer_SP)
  [M_MB] -> Add2/1
  Constant3/1 -> Force SP/5(rho_s_SP)
  [MB] -> Torque arm MB/1(MB)
  Selector2/1 -> Cross Product1/1
  Transpose3/1 -> [M_SP]
  Reshape1/1 -> S_B dot N_SP/1(N_SP)
  Areas_SP/1(A_vect) -> [A_vect_SP]
  Transpose1/1 -> [M_MB]
  Areas/1(A_vect) -> [A_vect]
  [P] -> Force MB/1(P)
  [S_B] -> S_B dot N_MB/2(S_B)
  [MB] -> Areas/1(MB)
  S_B dot N_MB/1(MB_illuminated) -> [NMB_true]
  [NMB_true] -> Force MB/2(NMB_true)
  N_MB/1 -> Reshape2/1
  MB/1 -> [MB]
  r_N/1 -> MatrixMultiply/2
  MatrixMultiply/1 -> Normalize Vector/1

== system pointing_group24/Desturbances/External Torques/SRP con frecce ==
  S_B : Inport
  Normalize Vector : vrlib/Utilities/Normalize Vector  maxzero=0
  SRP : Subsystem
  Tsrp : Outport
  wires:
  S_B/1 -> Normalize Vector/1
  Normalize Vector/1 -> SRP/1(S_B)
  SRP/1(Tsrp) -> Tsrp/1

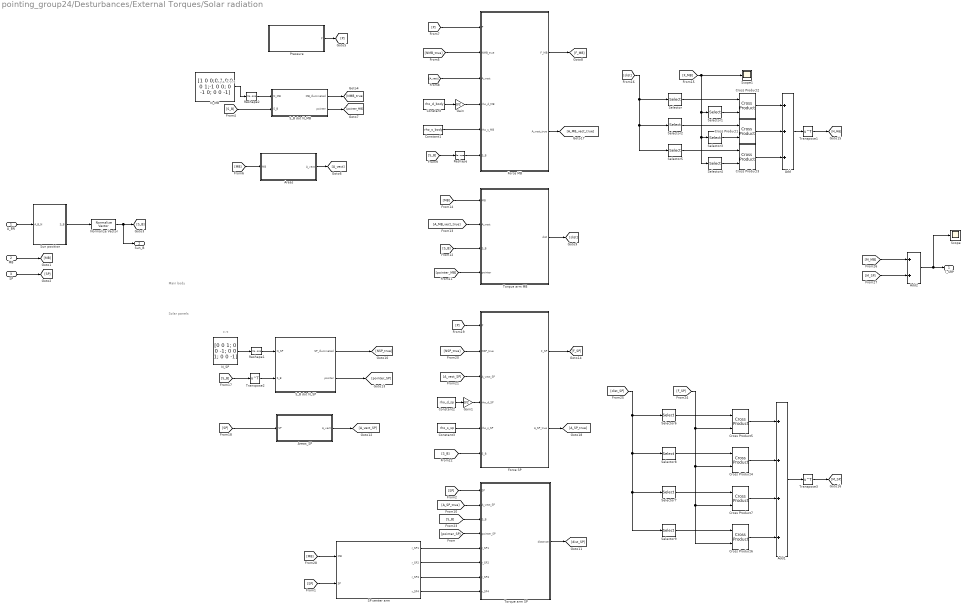
== system pointing_group24/Desturbances/External Torques/Solar radiation ==
  note: Main body
  note: x,y,z,-x,-y,-z
  note: z,-z
  note: Solar panels
  A_BN : Inport
  MB : Inport  Port=2
  SP : Inport  Port=3
  Add : Sum  Inputs=3
  Add1 : Sum  Inputs=++++
  Add2 : Sum
  Areas : Subsystem
  Areas_SP : Subsystem
  Constant : Constant  Value=rho_d_body
  Constant1 : Constant  Value=rho_s_body
  Constant2 : Constant  Value=rho_d_sp
  Constant3 : Constant  Value=rho_s_sp
  Cross Product{1..7} (7 alike) : matrix_library/Cross Product
  Force MB : Subsystem
  Force SP : Subsystem
  Gain : Gain  Gain=3/2
  Gain1 : Gain  Gain=3/2
  N_MB : Constant  Value=[1 0 0;0 1 0;0 0 1;-1 0 0; 0 -1 0; 0 0 -1]  VectorParams1D=off
  N_SP : Constant  Value=[0 0 1; 0 0 -1; 0 0 1; 0 0 -1]  VectorParams1D=off
  Normalize Vector : vrlib/Utilities/Normalize Vector  maxzero=0
  Pressure : Subsystem
  Reshape : Reshape  OutputDimensionality=Column vector (2-D)
  Reshape1 : Reshape  OutputDimensionality=Customize  OutputDimensions=[4,3]
  Reshape2 : Reshape  OutputDimensionality=Customize  OutputDimensions=[6,3]
  SP center arm : Subsystem
  S_B dot N_MB : Subsystem
  S_B dot N_SP : Subsystem
  Scope : Scope
  Scope1 : Scope
  Selector : Selector  NumberOfDimensions=2  InputPortWidth=3  IndexOptions=Index vector (dialog),Index vector (dialog)  Indices=1,[1 2 3]  OutputSizes=1,1
  Selector1 : Selector  NumberOfDimensions=2  InputPortWidth=3  IndexOptions=Index vector (dialog),Index vector (dialog)  Indices=1,[1 2 3]  OutputSizes=1,1
  Selector2 : Selector  NumberOfDimensions=2  InputPortWidth=3  IndexOptions=Index vector (dialog),Index vector (dialog)  Indices=2,[1 2 3]  OutputSizes=1,1
  Selector3 : Selector  NumberOfDimensions=2  InputPortWidth=3  IndexOptions=Index vector (dialog),Index vector (dialog)  Indices=2,[1 2 3]  OutputSizes=1,1
  Selector4 : Selector  NumberOfDimensions=2  InputPortWidth=3  IndexOptions=Index vector (dialog),Index vector (dialog)  Indices=3,[1 2 3]  OutputSizes=1,1
  Selector5 : Selector  NumberOfDimensions=2  InputPortWidth=3  IndexOptions=Index vector (dialog),Index vector (dialog)  Indices=3,[1 2 3]  OutputSizes=1,1
  Selector6 : Selector  NumberOfDimensions=2  InputPortWidth=3  IndexOptions=Index vector (dialog),Index vector (dialog)  Indices=1,[1 2 3]  OutputSizes=1,1
  Selector7 : Selector  NumberOfDimensions=2  InputPortWidth=3  IndexOptions=Index vector (dialog),Index vector (dialog)  Indices=3,[1 2 3]  OutputSizes=1,1
  Selector8 : Selector  NumberOfDimensions=2  InputPortWidth=3  IndexOptions=Index vector (dialog),Index vector (dialog)  Indices=2,[1 2 3]  OutputSizes=1,1
  Selector9 : Selector  NumberOfDimensions=2  InputPortWidth=3  IndexOptions=Index vector (dialog),Index vector (dialog)  Indices=4,[1 2 3]  OutputSizes=1,1
  Sun position : Subsystem
  Torque arm MB : Subsystem
  Torque arm SP : Subsystem
  Transpose1 : Math  Operator=transpose
  Transpose2 : Math  Operator=transpose
  Transpose3 : Math  Operator=transpose
  T_SRP : Outport
  Sun_B : Outport  Port=2
  wires:
  Sun position/1(S_B) -> Normalize Vector/1
  MB/1 -> [MB]
  N_MB/1 -> Reshape2/1
  [NMB_true] -> Force MB/2(NMB_true)
  S_B dot N_MB/1(MB_illuminated) -> [NMB_true]
  [MB] -> Areas/1(MB)
  [S_B] -> S_B dot N_MB/2(S_B)
  [P] -> Force MB/1(P)
  Areas/1(A_vect) -> [A_vect]
  Transpose1/1 -> [M_MB]
  Areas_SP/1(A_vect) -> [A_vect_SP]
  Reshape1/1 -> S_B dot N_SP/1(N_SP)
  Transpose3/1 -> [M_SP]
  Selector2/1 -> Cross Product1/1
  [MB] -> Torque arm MB/1(MB)
  Constant3/1 -> Force SP/5(rho_s_SP)
  [M_MB] -> Add2/1
  [pointer_SP] -> Torque arm SP/4(pointer_SP)
  Cross Product4/1 -> Add1/2
  [F_MB] -> Scope1/1, Selector4/1, Selector3/1, Selector1/1
  A_BN/1 -> Sun position/1(A_B_N)
  Add1/1 -> Transpose3/1
  Transpose2/1 -> S_B dot N_SP/2(S_B)
  [SP] -> Areas_SP/1(SP)
  [A_SP_true] -> Torque arm SP/2(A_vect_SP)
  Add/1 -> Transpose1/1
  Torque arm SP/1(distance) -> [dist_SP]
  Reshape2/1 -> S_B dot N_MB/1(N_MB)
  Torque arm MB/1(dist) -> [dist]
  S_B dot N_SP/2(pointer) -> [pointer_SP]
  Force MB/1(F_MB) -> [F_MB]
  Selector/1 -> Cross Product2/1
  [S_B] -> Reshape/1
  [P] -> Force SP/1(P)
  [A_vect] -> Force MB/3(A_vect)
  Selector1/1 -> Cross Product2/2
  Constant1/1 -> Force MB/5(rho_s_MB)
  [A_MB_vect_true] -> Torque arm MB/2(A_vect)
  Pressure/1(P) -> [P]
  Normalize Vector/1 -> Sun_B/1, [S_B]
  Constant2/1 -> Gain1/1
  Constant/1 -> Gain/1
  Selector8/1 -> Cross Product4/1
  [dist] -> Selector2/1, Selector5/1, Selector/1
  [NSP_true] -> Force SP/2(NSP_true)
  N_SP/1 -> Reshape1/1
  [S_B] -> Torque arm MB/3(S_B)
  Force SP/2(A_SP_true) -> [A_SP_true]
  [S_B] -> Torque arm SP/3(S_B)
  SP/1 -> [SP]
  Selector4/1 -> Cross Product3/2
  S_B dot N_MB/2(pointer) -> [pointer_MB]
  Force MB/2(A_vect_true) -> [A_MB_vect_true]
  [pointer_MB] -> Torque arm MB/4(pointer)
  Add2/1 -> Scope/1, T_SRP/1
  Selector3/1 -> Cross Product1/2
  [S_B] -> Force SP/6(S_B)
  [S_B] -> Transpose2/1
  Cross Product5/1 -> Add1/1
  [A_vect_SP] -> Force SP/3(A_vect_SP)
  Reshape/1 -> Force MB/6(S_B)
  Cross Product2/1 -> Add/1
  Force SP/1(F_SP) -> [F_SP]
  S_B dot N_SP/1(SP_illuminated) -> [NSP_true]
  Selector6/1 -> Cross Product5/1
  Selector5/1 -> Cross Product3/1
  Cross Product1/1 -> Add/2
  [M_SP] -> Add2/2
  [SP] -> Torque arm SP/1(SP)
  Cross Product3/1 -> Add/3
  [SP] -> SP center arm/2(SP)
  [MB] -> SP center arm/1(MB)
  SP center arm/1(r_SP1) -> Torque arm SP/5(r_SP1)
  SP center arm/2(r_SP2) -> Torque arm SP/6(r_SP2)
  Gain/1 -> Force MB/4(rho_d_MB)
  Gain1/1 -> Force SP/4(rho_d_SP)
  SP center arm/3(r_SP3) -> Torque arm SP/7(r_SP3)
  SP center arm/4(r_SP4) -> Torque arm SP/8(r_SP4)
  Selector7/1 -> Cross Product7/1
  Selector9/1 -> Cross Product6/1
  [dist_SP] -> Selector6/1, Selector9/1, Selector7/1, Selector8/1
  [F_SP] -> Cross Product5/2, Cross Product6/2, Cross Product7/2, Cross Product4/2
  Cross Product6/1 -> Add1/4
  Cross Product7/1 -> Add1/3

== system pointing_group24/Desturbances/External Torques/Sun position ==
  A_BN : Inport
  Clock : Clock
  Constant : Constant  Value=2*pi
  Constant1 : Constant  Value=365*24*3600
  Constant2 : Constant  Value=23.45
  Degrees to Radians : simulink_extras/Transformations/Degrees to Radians
  Divide : Product  Inputs=*/
  MatrixMultiply : Product  Multiplication=Matrix(*)
  Mux : Mux  Inputs=3
  Product1 : Product
  Product2 : Product
  Product3 : Product
  Reshape : Reshape  OutputDimensionality=Column vector (2-D)
  Sin : Trigonometry  Operator=cos
  Sin1 : Trigonometry
  Sin2 : Trigonometry  Operator=cos
  Sin3 : Trigonometry
  S_B : Outport
  wires:
  Product3/1 -> Mux/3
  Degrees to Radians/1 -> Sin3/1, Sin2/1
  Sin2/1 -> Product2/2
  Divide/1 -> Product1/1  "n"
  Constant2/1 -> Degrees to Radians/1
  Product1/1 -> Sin/1, Sin1/1  "theta_Sun"
  Product2/1 -> Mux/2
  Sin3/1 -> Product3/2
  Clock/1 -> Product1/2
  Sin1/1 -> Product3/1, Product2/1
  Constant/1 -> Divide/1
  Sin/1 -> Mux/1
  Constant1/1 -> Divide/2
  Mux/1 -> Reshape/1
  A_BN/1 -> MatrixMultiply/1
  MatrixMultiply/1 -> S_B/1
  Reshape/1 -> MatrixMultiply/2  "S_N"

== system pointing_group24/Desturbances/Orbital Mechanics/Sat Position magnitude ==
  note: 1+e cos(theta)
  note: a(1-e^2)
  note: Denominator
  note: Numerator
  theta : Inport
  Constant : Constant  Value=a
  Constant1 : Constant
  Constant3 : Constant  Value=e
  Constant4 : Constant
  Constant5 : Constant  Value=e
  Cos : Trigonometry  Operator=cos
  Divide : Product  Inputs=*/
  Product : Product
  Product1 : Product
  Square1 : Math  Operator=square
  Sum : Sum
  Sum1 : Sum  Inputs=+-
  r : Outport
  wires:
  Product1/1 -> Sum/1
  Sum1/1 -> Product/2
  Constant1/1 -> Sum1/1
  Sum/1 -> Divide/2
  Square1/1 -> Sum1/2
  Constant3/1 -> Product1/2
  Constant4/1 -> Sum/2
  Constant/1 -> Product/1
  Constant5/1 -> Square1/1
  Cos/1 -> Product1/1
  Product/1 -> Divide/1
  theta/1 -> Cos/1
  Divide/1 -> r/1

== system pointing_group24/Desturbances/Orbital Mechanics/Sat True Anomaly ==
  note: (1-e^2)^3/2
  note: n ( 1+e cos(theta))^2
  note: Denominator
  note: Numerator
  Constant : Constant  Value=n
  Constant1 : Constant
  Constant2 : Constant  Value=e
  Constant3 : Constant
  Constant4 : Constant  Value=e
  Constant5 : Constant  Value=3/2
  Cos : Trigonometry  Operator=cos
  Divide : Product  Inputs=*/
  Integrator : Integrator
  Power : Math  Operator=pow
  Product : Product
  Product1 : Product
  Square : Math  Operator=square
  Square1 : Math  Operator=square
  Sum : Sum
  Sum1 : Sum  Inputs=|+-
  theta : Outport
  wires:
  Sum/1 -> Square/1
  Integrator/1 -> theta/1, Cos/1  "theta"
  Square/1 -> Product1/2
  Constant5/1 -> Power/2
  Constant3/1 -> Sum1/1
  Product1/1 -> Divide/1
  Constant/1 -> Product1/1
  Divide/1 -> Integrator/1  "theta_dot"
  Square1/1 -> Sum1/2
  Product/1 -> Sum/2
  Power/1 -> Divide/2
  Constant1/1 -> Sum/1
  Constant2/1 -> Product/1
  Constant4/1 -> Square1/1
  Cos/1 -> Product/2
  Sum1/1 -> Power/1

== system pointing_group24/Desturbances/Orbital Mechanics/Sat pos & rel vel vectors in inertial frame ==
  note: r_N = r [cos(theta)
      | 		sin(theta)cos(i)
      | 		sin(theta)sin(i)]
  r : Inport
  theta : Inport  Port=2
  Constant : Constant  Value=2
  Constant1 : Constant
  Constant2 : Constant  Value=a
  Constant3 : Constant  Value=[0 0 om_E]
  Cos : Trigonometry  Operator=cos
  Cos1 : Trigonometry  Operator=cos
  Cross Product : matrix_library/Cross Product
  Divide : Product  Inputs=*/
  Divide1 : Product  Inputs=*/
  Gain : Gain  Gain=mu
  Orbit Inclination : Constant  Value=i
  Product{,1..3} (4 alike) : Product
  Sin : Trigonometry
  Sin1 : Trigonometry
  Sqrt : Sqrt
  Subtract : Sum  Inputs=-+
  Subtract1 : Sum  Inputs=+-
  Vector Concatenate : Concatenate  NumInputs=3  Mode=Multidimensional array
  r_N : Outport
  v_rel_N : Outport  Port=2
  wires:
  Sin/1 -> Product1/1, Product/1
  Product/1 -> Vector Concatenate/2
  Sin1/1 -> Product1/2
  r/1 -> Divide/2, Product2/1
  Orbit Inclination/1 -> Sin1/1, Cos1/1
  Vector Concatenate/1 -> Product3/2, Product2/2
  theta/1 -> Cos/1, Sin/1
  Cos/1 -> Vector Concatenate/1
  Cos1/1 -> Product/2
  Product1/1 -> Vector Concatenate/3
  Product2/1 -> Cross Product/2, r_N/1
  Constant/1 -> Divide/1
  Constant1/1 -> Divide1/1
  Constant2/1 -> Divide1/2
  Divide/1 -> Subtract/2
  Divide1/1 -> Subtract/1
  Subtract/1 -> Gain/1
  Gain/1 -> Sqrt/1
  Sqrt/1 -> Product3/1  "v"
  Product3/1 -> Subtract1/1  "v_N"
  Cross Product/1 -> Subtract1/2
  Constant3/1 -> Cross Product/1
  Subtract1/1 -> v_rel_N/1

== system pointing_group24/Desturbances/Relative Attitude/A_BL ==
  A_BN : Inport
  A_LN : Inport  Port=2
  Matrix Multiply : Product  Multiplication=Matrix(*)
  To Workspace : ToWorkspace  VariableName=A_BL  SampleTime=-1
  Transpose1 : matrix_library/Transpose
  A_BL : Outport
  wires:
  A_BN/1 -> Matrix Multiply/1
  A_LN/1 -> Transpose1/1
  Transpose1/1 -> Matrix Multiply/2
  Matrix Multiply/1 -> A_BL/1, To Workspace/1

== system pointing_group24/Desturbances/Relative Attitude/A_LN ==
  theta : Inport
  Constant : Constant  Value=0
  Constant1 : Constant  Value=[0; 0; 1]
  Constant2 : Constant  Value=[1 0 0; 0 cos(i) sin(i); 0 -sin(i) cos(i)]
  Cos : Trigonometry  Operator=cos
  Gain : Gain  Gain=[1; -1; 1]
  Matrix Concatenate : Concatenate  NumInputs=3  Mode=Multidimensional array  ConcatenateDimension=2
  Product : Product  Multiplication=Matrix(*)
  Selector : Selector  InputPortWidth=3  IndexOptions=Index vector (dialog)  Indices=[3 2 1]  OutputSizes=1
  Selector1 : Selector  InputPortWidth=3  IndexOptions=Index vector (dialog)  Indices=[2 3 1]  OutputSizes=1
  Sin : Trigonometry
  To Workspace : ToWorkspace  VariableName=A_LN  SampleTime=-1
  Vector Concatenate : Concatenate  NumInputs=3
  A_LN : Outport
  wires:
  Matrix Concatenate/1 -> Product/1
  theta/1 -> Sin/1, Cos/1
  Gain/1 -> Matrix Concatenate/1
  Vector Concatenate/1 -> Selector1/1, Selector/1
  Sin/1 -> Vector Concatenate/3
  Selector/1 -> Matrix Concatenate/2
  Selector1/1 -> Gain/1
  Product/1 -> A_LN/1, To Workspace/1
  Constant1/1 -> Matrix Concatenate/3
  Cos/1 -> Vector Concatenate/2
  Constant/1 -> Vector Concatenate/1
  Constant2/1 -> Product/2
